simulink model "pr4_simulink"  (R2024a)
settings: Solver=ode4  StartTime=0.0  StopTime=0.02  RelTol=1e-3
values from neighbouring files (symbols this model uses):
  A = [0 1; -1/(L*Cap) -R/L]    [pr4_pr1.m]    (also in pr4_prb3.m; pr4_pueb2.m)
  B = [0; 1/L]    [pr4_pr1.m]    (also in pr4_prb3.m; pr4_pueb2.m)
  C = [1 0]    [pr4_pr1.m]    (also in pr4_prb3.m; pr4_pueb2.m)
  D = 0    [pr4_pr1.m]    (also in pr4_prb3.m; pr4_pueb2.m)
settings Model: Creator=Monsty  LastModifiedBy=Monsty

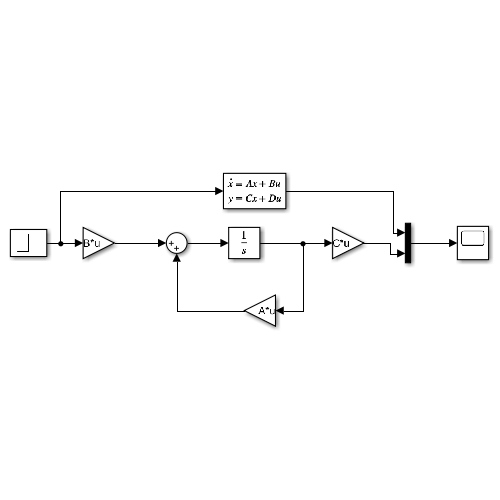
[thumbnail: Simulink's stored preview of the top-level diagram]
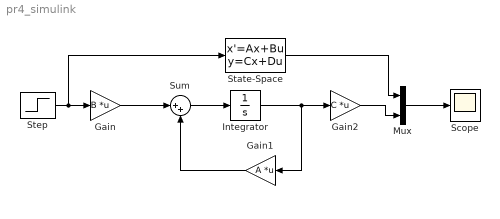
== system pr4_simulink ==
  Gain : Gain  Gain=B  Multiplication=Matrix(K*u)
  Gain1 : Gain  Gain=A  Multiplication=Matrix(K*u)
  Gain2 : Gain  Gain=C  Multiplication=Matrix(K*u)
  Integrator : Integrator
  Mux : Mux  Inputs=2
  Scope : Scope
  State-Space : StateSpace  A=A  B=B  C=C  D=D  InitialCondition=0
  Step : Step  Time=0.01  SampleTime=0
  Sum : Sum  Inputs=|++
  wires:
  Gain/1 -> Sum/1
  Gain1/1 -> Sum/2
  Step/1 -> State-Space/1, Gain/1
  Sum/1 -> Integrator/1
  Integrator/1 -> Gain1/1, Gain2/1
  State-Space/1 -> Mux/1
  Gain2/1 -> Mux/2
  Mux/1 -> Scope/1
